simulink model "full_system_nios_id7"  (R2021b)
settings: Solver=FixedStepDiscrete  StartTime=0.0  StopTime=250000  RelTol=1e-3
model workspace (MAT data in the model file):
  out_size = 0
undefined symbols (not defined in the file): betas, bias, DiscIntNeverNeededParam, mus, scale, sigmas
libraries: hdlsllib x2
settings Model: DataTypeOverride=Off  SimulationMode=accelerator  Creator=local_adm  LastModifiedBy=local_adm
settings SolverCC: AlgebraicLoopSolver=TrustRegion
settings DataIOCC: LimitDataPoints=on  SaveOutput=off  SaveTime=off
settings OptimizationCC: BlockReduction=off  ConditionallyExecuteInputs=off  DefaultParameterBehavior=Inlined  LifeSpan=inf
settings DebuggingCC: AlgebraicLoopMsg=error  SingleTaskRateTransMsg=error  ParameterPrecisionLossMsg=none  AllowSymbolicDim=off  StrictBusMsg=ErrorOnBusTreatedAsVector  SFUnexpectedBacktrackingDiag=warning  SFNoUnconditionalDefaultTransitionDiag=warning  SFExecutionAtInitializationDiag=none  SFMachineParentedDataDiag=warning  ArithmeticOperatorsInVariantConditions=warning
settings HardwareCC: ProdBitPerPointer=32  ProdBitPerSizeT=32  ProdBitPerPtrDiffT=32  ProdLargestAtomicFloat=None  ProdIntDivRoundTo=Undefined  ProdEndianess=Unspecified  ProdWordSize=32  ProdHWDeviceType=ASIC/FPGA->ASIC/FPGA  ProdEqTarget=off
settings SFSimCC: SimUseLocalCustomCode=off  CustomCodeUndefinedFunction=UseInterfaceOnly
settings RTWCC: RTWUseLocalCustomCode=off
settings CodeAppCC: StateflowObjectComments=on
settings GRTTargetCC: TargetLangStandard=C89/C90 (ANSI)
settings ConfigComp: CovScope=ReferencedModels  CovMetricSettings=dw  CovSaveCumulativeToWorkspaceVar=on  CovSaveSingleToWorkspaceVar=on  CovExternalEMLEnable=off  CovSFcnEnable=off

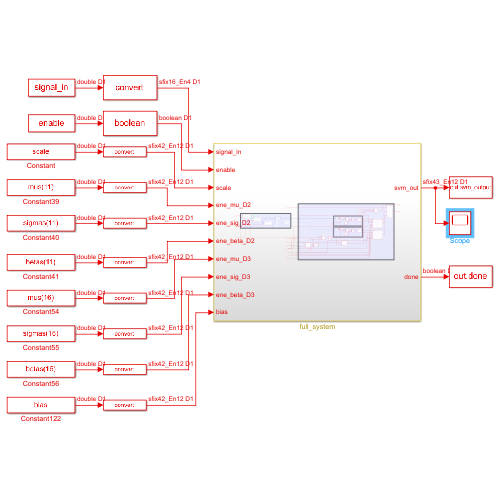
[thumbnail: Simulink's stored preview of the top-level diagram]
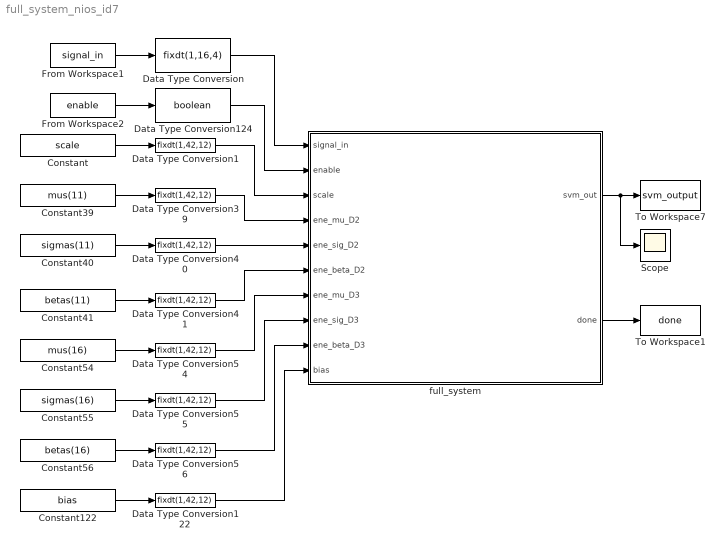
== system full_system_nios_id7 ==
  Constant : Constant  Value=scale  VectorParams1D=off  SampleTime=-1
  Constant122 : Constant  Value=bias  VectorParams1D=off  SampleTime=-1
  Constant39 : Constant  Value=mus(11)  VectorParams1D=off  SampleTime=-1
  Constant40 : Constant  Value=sigmas(11)  VectorParams1D=off  SampleTime=-1
  Constant41 : Constant  Value=betas(11)  VectorParams1D=off  SampleTime=-1
  Constant54 : Constant  Value=mus(16)  VectorParams1D=off  SampleTime=-1
  Constant55 : Constant  Value=sigmas(16)  VectorParams1D=off  SampleTime=-1
  Constant56 : Constant  Value=betas(16)  VectorParams1D=off  SampleTime=-1
  Data Type Conversion : DataTypeConversion  OutMax=2  OutDataTypeStr=fixdt(1,16,4)
  Data Type Conversion{1,39..41,54..56,122} (8 alike) : DataTypeConversion  OutMax=2  OutDataTypeStr=fixdt(1,42,12)
  Data Type Conversion124 : DataTypeConversion  OutMax=1  OutDataTypeStr=boolean
  From Workspace1 : FromWorkspace  VariableName=signal_in  SampleTime=1  OutputAfterFinalValue=Setting to zero
  From Workspace2 : FromWorkspace  VariableName=enable  SampleTime=1  OutputAfterFinalValue=Setting to zero
  Scope : Scope
  To Workspace1 : ToWorkspace  VariableName=done  SampleTime=-1
  To Workspace7 : ToWorkspace  VariableName=svm_output  SampleTime=-1
  full_system : Subsystem
  wires:
  Data Type Conversion41/1 -> full_system/6(ene_beta_D2)
  Data Type Conversion56/1 -> full_system/9(ene_beta_D3)
  From Workspace2/1 -> Data Type Conversion124/1
  full_system/2(done) -> To Workspace1/1
  Data Type Conversion122/1 -> full_system/10(bias)
  Data Type Conversion55/1 -> full_system/8(ene_sig_D3)
  Data Type Conversion54/1 -> full_system/7(ene_mu_D3)
  Data Type Conversion40/1 -> full_system/5(ene_sig_D2)
  Data Type Conversion39/1 -> full_system/4(ene_mu_D2)
  Data Type Conversion1/1 -> full_system/3(scale)
  Data Type Conversion124/1 -> full_system/2(enable)
  Data Type Conversion/1 -> full_system/1(signal_in)
  Constant122/1 -> Data Type Conversion122/1
  Constant56/1 -> Data Type Conversion56/1
  Constant54/1 -> Data Type Conversion54/1
  Constant55/1 -> Data Type Conversion55/1
  Constant41/1 -> Data Type Conversion41/1
  Constant39/1 -> Data Type Conversion39/1
  Constant40/1 -> Data Type Conversion40/1
  Constant/1 -> Data Type Conversion1/1
  From Workspace1/1 -> Data Type Conversion/1
  full_system/1(svm_out) -> Scope/1, To Workspace7/1

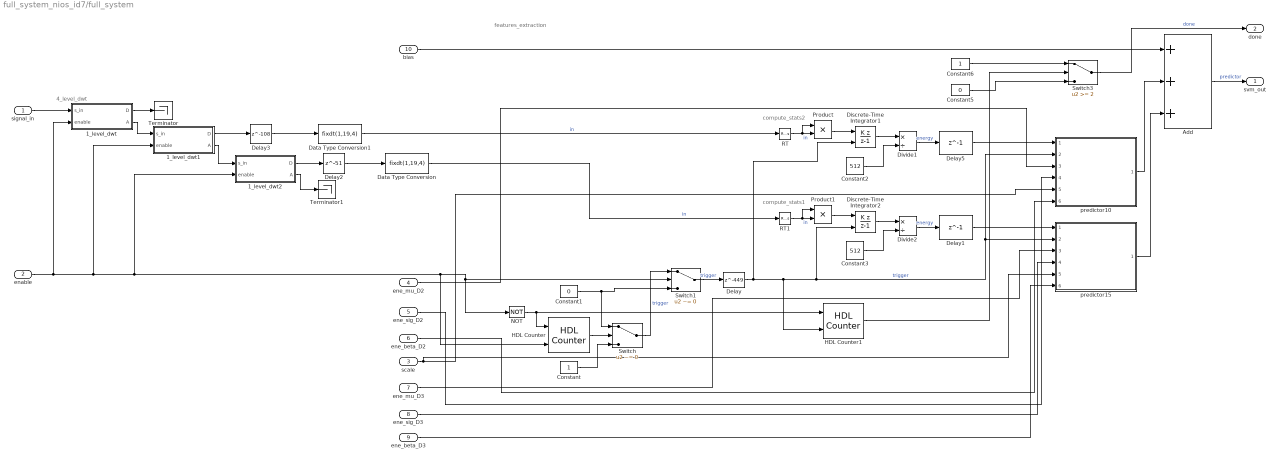
== system full_system_nios_id7/full_system ==
  note: 4_level_dwt
  note: features_extraction
  note: compute_stats2
  note: compute_stats1
  signal_in : Inport
  enable : Inport  Port=2
  scale : Inport  Port=3
  ene_mu_D2 : Inport  Port=4
  ene_sig_D2 : Inport  Port=5
  ene_beta_D2 : Inport  Port=6
  ene_mu_D3 : Inport  Port=7
  ene_sig_D3 : Inport  Port=8
  ene_beta_D3 : Inport  Port=9
  bias : Inport  Port=10
  1_level_dwt : Subsystem
  1_level_dwt1 : Subsystem
  1_level_dwt2 : Subsystem
  Add : Sum  Inputs=+++
  Constant : Constant  VectorParams1D=off  OutDataTypeStr=boolean  SampleTime=-1
  Constant1 : Constant  Value=0  VectorParams1D=off  OutDataTypeStr=boolean  SampleTime=-1
  Constant2 : Constant  Value=512  VectorParams1D=off  OutDataTypeStr=uint16  SampleTime=-1
  Constant3 : Constant  Value=512  VectorParams1D=off  OutDataTypeStr=uint16  SampleTime=-1
  Constant5 : Constant  Value=0  VectorParams1D=off  OutDataTypeStr=boolean  SampleTime=-1
  Constant6 : Constant  VectorParams1D=off  OutDataTypeStr=boolean  SampleTime=-1
  Data Type Conversion : DataTypeConversion  OutDataTypeStr=fixdt(1,19,4)
  Data Type Conversion1 : DataTypeConversion  OutDataTypeStr=fixdt(1,19,4)
  Delay : Delay  DelayLength=449  InitialCondition=0  UseCircularBuffer=on
  Delay1 : Delay  DelayLength=1  InitialCondition=0  UseCircularBuffer=on
  Delay2 : Delay  DelayLength=51
  Delay3 : Delay  DelayLength=108
  Delay5 : Delay  DelayLength=1  InitialCondition=0  UseCircularBuffer=on
  Discrete-Time Integrator1 : DiscreteIntegrator  IntegratorMethod=Accumulation: Backward Euler  ExternalReset=rising  SampleTime=-1  ICPrevOutput=DiscIntNeverNeededParam  ICPrevScaledInput=DiscIntNeverNeededParam
  Discrete-Time Integrator2 : DiscreteIntegrator  IntegratorMethod=Accumulation: Backward Euler  ExternalReset=rising  SampleTime=-1  ICPrevOutput=DiscIntNeverNeededParam  ICPrevScaledInput=DiscIntNeverNeededParam
  Divide1 : Product  Inputs=*/  RndMeth=Zero  SaturateOnIntegerOverflow=on
  Divide2 : Product  Inputs=*/  RndMeth=Zero  SaturateOnIntegerOverflow=on
  HDL Counter : hdlsllib/Sources/HDL Counter  CountType=Count limited  CountInit=0  CountStep=1  CountMax=511  CountFromType=Initial value  CountFrom=0  CountResetPort=on  CountLoadPort=off  CountEnbPort=on  CountDirPort=off  CountHitOutputPort=off  CountDataType=Unsigned  CountWordLen=9  CountFracLen=0  CountSampTime=1
  HDL Counter1 : hdlsllib/Sources/HDL Counter  CountType=Count limited  CountInit=0  CountStep=1  CountMax=2  CountFromType=Initial value  CountFrom=0  CountResetPort=on  CountLoadPort=off  CountEnbPort=on  CountDirPort=off  CountHitOutputPort=off  CountDataType=Unsigned  CountWordLen=4  CountFracLen=0  CountSampTime=1
  NOT : Logic  Operator=NOT  IconShape=distinctive  AllPortsSameDT=off  OutDataTypeStr=boolean
  Product : Product
  Product1 : Product
  RT : RateTransition  OutPortSampleTime=1
  RT1 : RateTransition  OutPortSampleTime=1
  Switch : Switch  Criteria=u2 ~= 0
  Switch1 : Switch  Criteria=u2 ~= 0
  Switch3 : Switch  Threshold=2
  Terminator : Terminator
  Terminator1 : Terminator
  predictor10 : Subsystem  ReferencedSubsystem=predictor_2021b
  predictor15 : Subsystem  ReferencedSubsystem=predictor_2021b
  svm_out : Outport
  done : Outport  Port=2
  wires:
  RT1/1 -> Product1/2, Product1/1  "in"
  Constant5/1 -> Switch3/3
  Product/1 -> Discrete-Time Integrator1/1
  predictor15/1 -> Add/3
  Switch1/1 -> Delay/1  "trigger"
  enable/1 -> Switch1/2, NOT/1, HDL Counter/2, 1_level_dwt2/2(enable), 1_level_dwt1/2(enable), 1_level_dwt/2(enable)
  scale/1 -> predictor10/5, predictor15/5
  Constant/1 -> Switch/3
  HDL Counter1/1 -> Switch3/2
  Constant3/1 -> Divide2/2
  Product1/1 -> Discrete-Time Integrator2/1
  Constant6/1 -> Switch3/1
  predictor10/1 -> Add/2
  HDL Counter/1 -> Switch/2
  Constant1/1 -> Switch1/3, Switch/1
  Switch/1 -> Switch1/1  "trigger"
  NOT/1 -> HDL Counter1/1, HDL Counter/1
  Delay/1 -> predictor10/2, predictor15/2, Discrete-Time Integrator2/2, HDL Counter1/2, Discrete-Time Integrator1/2  "trigger"
  Divide1/1 -> Delay5/1  "energy"
  Divide2/1 -> Delay1/1  "energy"
  Discrete-Time Integrator2/1 -> Divide2/1
  1_level_dwt1/1(D) -> Delay3/1
  1_level_dwt2/2(A) -> Terminator1/1
  Discrete-Time Integrator1/1 -> Divide1/1
  Constant2/1 -> Divide1/2
  RT/1 -> Product/2, Product/1  "in"
  Delay3/1 -> Data Type Conversion1/1
  1_level_dwt/1(D) -> Terminator/1
  Delay2/1 -> Data Type Conversion/1
  1_level_dwt2/1(D) -> Delay2/1
  1_level_dwt1/2(A) -> 1_level_dwt2/1(s_in)
  1_level_dwt/2(A) -> 1_level_dwt1/1(s_in)
  signal_in/1 -> 1_level_dwt/1(s_in)
  bias/1 -> Add/1
  ene_sig_D3/1 -> predictor15/4
  ene_beta_D2/1 -> predictor10/6
  ene_sig_D2/1 -> predictor10/4
  ene_mu_D2/1 -> predictor10/3
  ene_mu_D3/1 -> predictor15/3
  ene_beta_D3/1 -> predictor15/6
  Add/1 -> svm_out/1  "predictor"
  Switch3/1 -> done/1  "done"
  Delay1/1 -> predictor15/1
  Delay5/1 -> predictor10/1
  Data Type Conversion1/1 -> RT/1  "in"
  Data Type Conversion/1 -> RT1/1  "in"

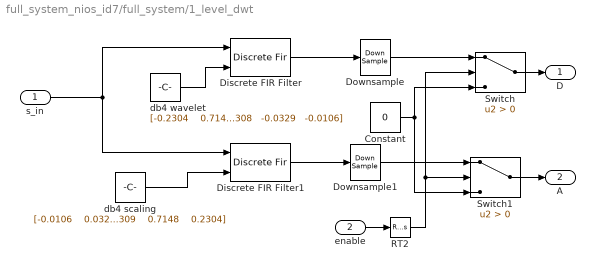
== system full_system_nios_id7/full_system/1_level_dwt ==
  s_in : Inport
  enable : Inport  Port=2
  Constant : Constant  Value=0  OutDataTypeStr=Inherit: Inherit via back propagation  SampleTime=-1
  Discrete FIR Filter : DiscreteFir  CoefSource=Input port
      settings: InputPortMap=u0,u1
  Discrete FIR Filter1 : DiscreteFir  CoefSource=Input port
      settings: InputPortMap=u0,u1
  Downsample : DownSample  phase=1  RateOptions=Allow multirate processing
  Downsample1 : DownSample  phase=1  RateOptions=Allow multirate processing
  RT2 : RateTransition  OutPortSampleTime=2
  Switch : Switch  Criteria=u2 > Threshold
  Switch1 : Switch  Criteria=u2 > Threshold
  db4 scaling : Constant  Value="[-0.0106    0.0329    0.0308   -0.1870   -0.0280    0.6309    0.7148    0.2304]"  OutDataTypeStr=Inherit: Inherit via back propagation  SampleTime=-1
  db4 wavelet : Constant  Value="[-0.2304    0.7148   -0.6309   -0.0280    0.1870    0.0308   -0.0329   -0.0106]"  OutDataTypeStr=Inherit: Inherit via back propagation  SampleTime=-1
  D : Outport
  A : Outport  Port=2
  wires:
  db4 wavelet/1 -> Discrete FIR Filter/2
  s_in/1 -> Discrete FIR Filter1/1, Discrete FIR Filter/1
  db4 scaling/1 -> Discrete FIR Filter1/2
  Constant/1 -> Switch/3, Switch1/3
  Discrete FIR Filter/1 -> Downsample/1
  Discrete FIR Filter1/1 -> Downsample1/1
  Switch1/1 -> A/1
  Switch/1 -> D/1
  Downsample/1 -> Switch/1
  Downsample1/1 -> Switch1/1
  enable/1 -> RT2/1
  RT2/1 -> Switch/2, Switch1/2

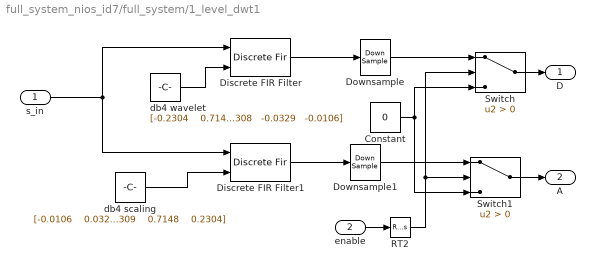
== system full_system_nios_id7/full_system/1_level_dwt1 ==
  s_in : Inport
  enable : Inport  Port=2
  Constant : Constant  Value=0  OutDataTypeStr=Inherit: Inherit via back propagation  SampleTime=-1
  Discrete FIR Filter : DiscreteFir  CoefSource=Input port
      settings: InputPortMap=u0,u1
  Discrete FIR Filter1 : DiscreteFir  CoefSource=Input port
      settings: InputPortMap=u0,u1
  Downsample : DownSample  phase=1  RateOptions=Allow multirate processing
  Downsample1 : DownSample  phase=1  RateOptions=Allow multirate processing
  RT2 : RateTransition  OutPortSampleTime=4
  Switch : Switch  Criteria=u2 > Threshold
  Switch1 : Switch  Criteria=u2 > Threshold
  db4 scaling : Constant  Value="[-0.0106    0.0329    0.0308   -0.1870   -0.0280    0.6309    0.7148    0.2304]"  OutDataTypeStr=Inherit: Inherit via back propagation  SampleTime=-1
  db4 wavelet : Constant  Value="[-0.2304    0.7148   -0.6309   -0.0280    0.1870    0.0308   -0.0329   -0.0106]"  OutDataTypeStr=Inherit: Inherit via back propagation  SampleTime=-1
  D : Outport
  A : Outport  Port=2
  wires:
  db4 wavelet/1 -> Discrete FIR Filter/2
  s_in/1 -> Discrete FIR Filter1/1, Discrete FIR Filter/1
  db4 scaling/1 -> Discrete FIR Filter1/2
  Constant/1 -> Switch/3, Switch1/3
  Discrete FIR Filter/1 -> Downsample/1
  Discrete FIR Filter1/1 -> Downsample1/1
  Switch1/1 -> A/1
  Switch/1 -> D/1
  Downsample/1 -> Switch/1
  Downsample1/1 -> Switch1/1
  enable/1 -> RT2/1
  RT2/1 -> Switch/2, Switch1/2

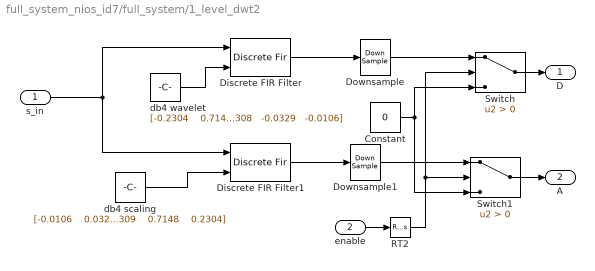
== system full_system_nios_id7/full_system/1_level_dwt2 ==
  s_in : Inport
  enable : Inport  Port=2
  Constant : Constant  Value=0  OutDataTypeStr=Inherit: Inherit via back propagation  SampleTime=-1
  Discrete FIR Filter : DiscreteFir  CoefSource=Input port
      settings: InputPortMap=u0,u1
  Discrete FIR Filter1 : DiscreteFir  CoefSource=Input port
      settings: InputPortMap=u0,u1
  Downsample : DownSample  phase=1  RateOptions=Allow multirate processing
  Downsample1 : DownSample  phase=1  RateOptions=Allow multirate processing
  RT2 : RateTransition  OutPortSampleTime=8
  Switch : Switch  Criteria=u2 > Threshold
  Switch1 : Switch  Criteria=u2 > Threshold
  db4 scaling : Constant  Value="[-0.0106    0.0329    0.0308   -0.1870   -0.0280    0.6309    0.7148    0.2304]"  OutDataTypeStr=Inherit: Inherit via back propagation  SampleTime=-1
  db4 wavelet : Constant  Value="[-0.2304    0.7148   -0.6309   -0.0280    0.1870    0.0308   -0.0329   -0.0106]"  OutDataTypeStr=Inherit: Inherit via back propagation  SampleTime=-1
  D : Outport
  A : Outport  Port=2
  wires:
  db4 wavelet/1 -> Discrete FIR Filter/2
  s_in/1 -> Discrete FIR Filter1/1, Discrete FIR Filter/1
  db4 scaling/1 -> Discrete FIR Filter1/2
  Constant/1 -> Switch/3, Switch1/3
  Discrete FIR Filter/1 -> Downsample/1
  Discrete FIR Filter1/1 -> Downsample1/1
  Switch1/1 -> A/1
  Switch/1 -> D/1
  Downsample/1 -> Switch/1
  Downsample1/1 -> Switch1/1
  enable/1 -> RT2/1
  RT2/1 -> Switch/2, Switch1/2
